simulink model "exam2021_sat"  (R2021b)
settings: Solver=VariableStepAuto  StartTime=0.0  StopTime=50  RelTol=1e-3
settings Model: Creator=rohan  LastModifiedBy=rohan

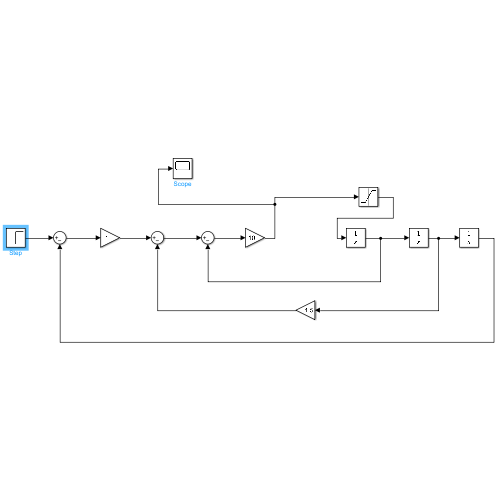
[thumbnail: Simulink's stored preview of the top-level diagram]
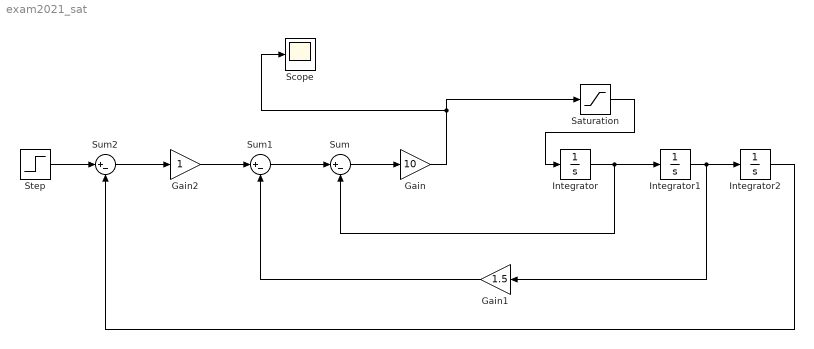
== system exam2021_sat ==
  Gain : Gain  Gain=10
  Gain1 : Gain  Gain=1.5
  Gain2 : Gain
  Integrator : Integrator
  Integrator1 : Integrator
  Integrator2 : Integrator
  Saturation : Saturate
  Scope : Scope
  Step : Step  After=1.5061  SampleTime=0
  Sum : Sum  Inputs=|+-
  Sum1 : Sum  Inputs=|+-
  Sum2 : Sum  Inputs=|+-
  wires:
  Gain/1 -> Saturation/1, Scope/1
  Sum/1 -> Gain/1
  Integrator/1 -> Integrator1/1, Sum/2
  Integrator1/1 -> Gain1/1, Integrator2/1
  Sum1/1 -> Sum/1
  Gain1/1 -> Sum1/2
  Gain2/1 -> Sum1/1
  Sum2/1 -> Gain2/1
  Integrator2/1 -> Sum2/2
  Step/1 -> Sum2/1
  Saturation/1 -> Integrator/1
